simulink model "spacecraft4_2"  (R2019b)
settings: Solver=VariableStepAuto  StartTime=0.0  StopTime=10.0  RelTol=1e-3
values from neighbouring files (symbols this model uses):
  K = lqr(A,B,Q,R)    [LQG_calcs.m]
undefined symbols (not defined in the file or in its folder): Discrete, Time
libraries: ctrlSharedLib x1
settings Model: Creator=Tesla  LastModifiedBy=Tesla

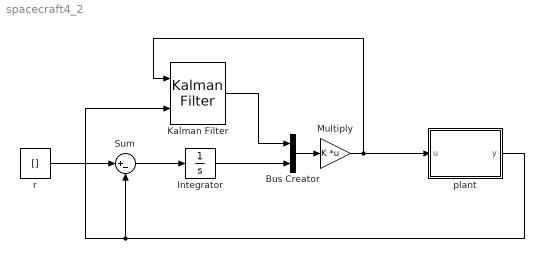
== system spacecraft4_2 ==
  Bus Creator : BusCreator  Inputs=2
  Integrator : Integrator
  Kalman Filter : ctrlSharedLib/Kalman Filter  TimeDomain=Discrete-Time  UseCurrentEstimator=on  ModelSource=LTI State-Space Variable  ModelSourceVariable=ss(0.95,1,1,0,1)  A=0.95  B=1  C=1  D=0  NumberOfStates=1  NumberOfInputs=1  NumberOfOutputs=1  InitialEstimateSource=Dialog  X0=0  P0=10  UseK=off  UseGH=off  NumberOfProcessNoiseInputs=1  G=1  TimeInvariantG=on  H=0  TimeInvariantH=on  Q=0.05  TimeInvariantQ=on  R=1  TimeInvariantR=on  N=0  TimeInvariantN=on  AddInputPort=on  AddEnablePort=off  OutputEstimatedY=off  OutputP=off  Ts=-1
      settings: SourceProductBaseCode=CT
  Multiply : Gain  Gain=K  Multiplication=Matrix(K*u) (u vector)
  Sum : Sum  Inputs=|+-
  "plant " : MATLAB Function  TreatAsAtomicUnit=on
  r : Constant  Value=[]
  wires:
  r/1 -> Sum/1
  "plant "/1(y) -> Kalman Filter/2, Sum/2
  Sum/1 -> Integrator/1
  Multiply/1 -> "plant "/1(u), Kalman Filter/1
  Kalman Filter/1 -> Bus Creator/1
  Bus Creator/1 -> Multiply/1
  Integrator/1 -> Bus Creator/2

== matlab function spacecraft4_2/plant  ==
  data: u input; y output
function y = fcn(u)

y = u;
